simulink model "voter_logic_harness"  (Simulink 8.7)
settings: Solver=FixedStepDiscrete  StartTime=0  StopTime=1  FixedStep=1  RelTol=1e-3
undefined symbols (not defined in the file or in its folder): sigbuilder_block
libraries: sldvlib x10, simulink x6
settings Model: SldvGeneratedHarnessModel=TestUnitModel=voter_logic|
settings DataIOCC: SaveFormat=StructureWithTime
settings OptimizationCC: BlockReduction=off  ExpressionFolding=off
settings DebuggingCC: UnderspecifiedInitializationDetection=Simplified  MergeDetectMultiDrivingBlocksExec=error  InheritedTsInSrcMsg=none  AllowSymbolicDim=off
settings HardwareCC: ProdBitPerPointer=64  ProdLargestAtomicFloat=Float  ProdIntDivRoundTo=Zero  ProdEndianess=LittleEndian  ProdWordSize=64  ProdHWDeviceType=Intel->x86-64 (Windows64)
settings GRTTargetCC: GeneratePreprocessorConditionals=Use local settings
settings ConfigComp: CovModelRefEnable=off

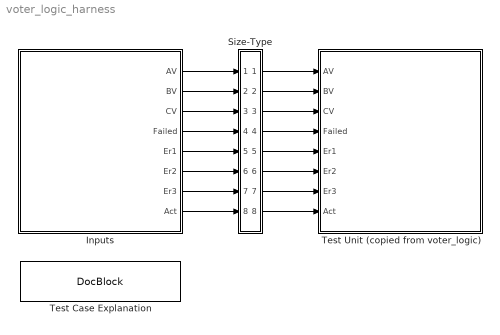
== system voter_logic_harness ==
  Inputs : Subsystem  Tag=STV Subsys  LoadFcn=sigbuilder_block('load',[459.75 78 519.75 399.75 ]);  StartFcn=sigbuilder_block('start');  StopFcn=sigbuilder_block('stop');  ClipboardFcn=sigbuilder_block('clipboard');  mask(Sigbuilder block){}
      mask init:
      | if ~strcmp(get_param(bdroot(gcb),'SimulationStatus'),'stopped'),tuvar = sigbuilder_block('maskInit'); end
      settings: CopyFcn=sigbuilder_block('copy');  DeleteFcn=sigbuilder_block('delete');  ModelCloseFcn=sigbuilder_block('modelClose');  PreSaveFcn=sigbuilder_block('preSave');  PauseFcn=sigbuilder_block('pause');  ContinueFcn=sigbuilder_block('continue');  NameChangeFcn=sigbuilder_block('namechange');  OpenFcn=sigbuilder_block('open');  CloseFcn=sigbuilder_block('close');
      mask Display: plot(0, 0, 100, 100,[2, 2, 32, 32, 2], [68, 8, 8, 68, 68],[32, 2], [38, 38], [32, 19, 2],[53, 60, 44], [32, 17, 17, 2],[16, 16, 31, 31]);txt = getActiveGroup(gcbh);text(2, 100, txt,'verticalAlignment', 'top');
  Size-Type : Subsystem
  Test Case Explanation : simulink/Model-Wide Utilities/DocBlock  DocumentType=Text
  Test Unit (copied from voter_logic) : Subsystem
  wires:
  Inputs/1(AV) -> Size-Type/1(In1)
  Size-Type/1(Out1) -> Test Unit (copied from voter_logic)/1(AV)
  Inputs/2(BV) -> Size-Type/2(In2)
  Size-Type/2(Out2) -> Test Unit (copied from voter_logic)/2(BV)
  Inputs/3(CV) -> Size-Type/3(In3)
  Size-Type/3(Out3) -> Test Unit (copied from voter_logic)/3(CV)
  Inputs/4(Failed) -> Size-Type/4(In4)
  Size-Type/4(Out4) -> Test Unit (copied from voter_logic)/4(Failed)
  Inputs/5(Er1) -> Size-Type/5(In5)
  Size-Type/5(Out5) -> Test Unit (copied from voter_logic)/5(Er1)
  Inputs/6(Er2) -> Size-Type/6(In6)
  Size-Type/6(Out6) -> Test Unit (copied from voter_logic)/6(Er2)
  Inputs/7(Er3) -> Size-Type/7(In7)
  Size-Type/7(Out7) -> Test Unit (copied from voter_logic)/7(Er3)
  Inputs/8(Act) -> Size-Type/8(In8)
  Size-Type/8(Out8) -> Test Unit (copied from voter_logic)/8(Act)

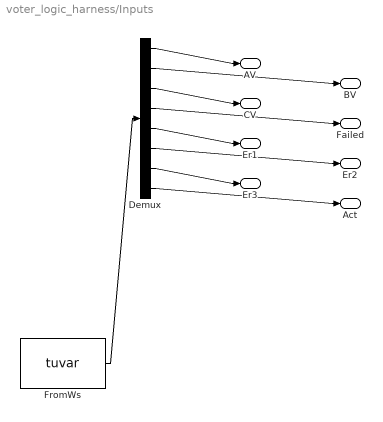
== system voter_logic_harness/Inputs ==
  Demux : Demux  Tag=STV Demux  Outputs=8
  FromWs : FromWorkspace  Tag=STV FromWs  VariableName=tuvar  SampleTime=0  SigBuilderData=DataTag0  VnvData=DataTag1
      SigBuilderData=|
      | dataSet.timeRange = [0 1]
      | dataSet.name = 'Counterexample 1'
      | sbobj.Name = 'Signal Builder'
      | sbobj.Groups.Name = 'Counterexample 1'
      | sbobj.Groups.Signals(1).Name = 'AV'
      | sbobj.Groups.Signals(1).XData = [0 1]
      | sbobj.Groups.Signals(1).YData = [1 1]
      | sbobj.Groups.Signals(2).Name = 'BV'
      | sbobj.Groups.Signals(2).XData = [0 1]
      | sbobj.Groups.Signals(2).YData = [0 0]
      | sbobj.Groups.Signals(3).Name = 'CV'
      | sbobj.Groups.Signals(3).XData = [0 1]
      | sbobj.Groups.Signals(3).YData = [1 1]
      | sbobj.Groups.Signals(4).Name = 'Failed'
      | sbobj.Groups.Signals(4).XData = [0 1]
      | sbobj.Groups.Signals(4).YData = [3 3]
      | sbobj.Groups.Signals(5).Name = 'Er1'
      | sbobj.Groups.Signals(5).XData = [0 1]
      | sbobj.Groups.Signals(5).YData = [-3 -3]
      | sbobj.Groups.Signals(6).Name = 'Er2'
      | sbobj.Groups.Signals(6).XData = [0 1]
      | sbobj.Groups.Signals(6).YData = [-3 -3]
      | sbobj.Groups.Signals(7).Name = 'Er3'
      | sbobj.Groups.Signals(7).XData = [0 1]
      | sbobj.Groups.Signals(7).YData = [-9 -9]
      | sbobj.Groups.Signals(8).Name = 'Act'
      | sbobj.Groups.Signals(8).XData = [0 1]
      | sbobj.Groups.Signals(8).YData = [60 60]
      | sbobj.Groups.TimeRange = [0 1]
  AV : Outport  Tag=STV Outport
  BV : Outport  Tag=STV Outport  Port=2
  CV : Outport  Tag=STV Outport  Port=3
  Failed : Outport  Tag=STV Outport  Port=4
  Er1 : Outport  Tag=STV Outport  Port=5
  Er2 : Outport  Tag=STV Outport  Port=6
  Er3 : Outport  Tag=STV Outport  Port=7
  Act : Outport  Tag=STV Outport  Port=8
  wires:
  FromWs/1 -> Demux/1
  Demux/1 -> AV/1
  Demux/2 -> BV/1
  Demux/3 -> CV/1
  Demux/4 -> Failed/1
  Demux/5 -> Er1/1
  Demux/6 -> Er2/1
  Demux/7 -> Er3/1
  Demux/8 -> Act/1

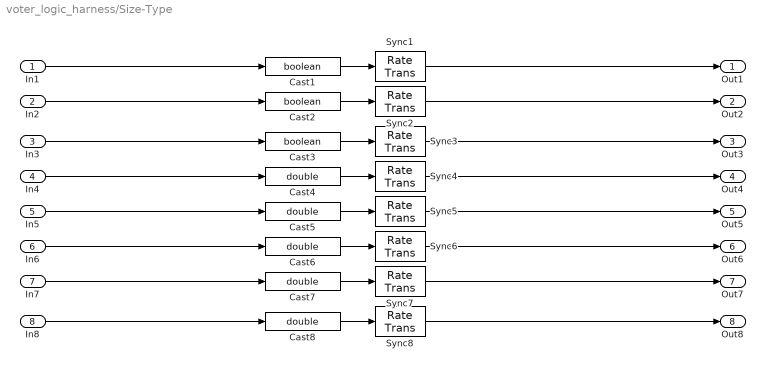
== system voter_logic_harness/Size-Type ==
  In1 : Inport
  In2 : Inport  Port=2
  In3 : Inport  Port=3
  In4 : Inport  Port=4
  In5 : Inport  Port=5
  In6 : Inport  Port=6
  In7 : Inport  Port=7
  In8 : Inport  Port=8
  Cast1 : DataTypeConversion  OutDataTypeStr=boolean  RndMeth=Nearest  SaturateOnIntegerOverflow=on
  Cast2 : DataTypeConversion  OutDataTypeStr=boolean  RndMeth=Nearest  SaturateOnIntegerOverflow=on
  Cast3 : DataTypeConversion  OutDataTypeStr=boolean  RndMeth=Nearest  SaturateOnIntegerOverflow=on
  Cast{4..8} (5 alike) : DataTypeConversion  OutDataTypeStr=double  RndMeth=Nearest  SaturateOnIntegerOverflow=on
  Sync{1..8} (8 alike) : RateTransition  OutPortSampleTime=[1,0]
  Out1 : Outport
  Out2 : Outport  Port=2
  Out3 : Outport  Port=3
  Out4 : Outport  Port=4
  Out5 : Outport  Port=5
  Out6 : Outport  Port=6
  Out7 : Outport  Port=7
  Out8 : Outport  Port=8
  wires:
  In1/1 -> Cast1/1
  Cast1/1 -> Sync1/1
  Sync1/1 -> Out1/1
  In2/1 -> Cast2/1
  Cast2/1 -> Sync2/1
  Sync2/1 -> Out2/1
  In3/1 -> Cast3/1
  Cast3/1 -> Sync3/1
  Sync3/1 -> Out3/1
  In4/1 -> Cast4/1
  Cast4/1 -> Sync4/1
  Sync4/1 -> Out4/1
  In5/1 -> Cast5/1
  Cast5/1 -> Sync5/1
  Sync5/1 -> Out5/1
  In6/1 -> Cast6/1
  Cast6/1 -> Sync6/1
  Sync6/1 -> Out6/1
  In7/1 -> Cast7/1
  Cast7/1 -> Sync7/1
  Sync7/1 -> Out7/1
  In8/1 -> Cast8/1
  Cast8/1 -> Sync8/1
  Sync8/1 -> Out8/1

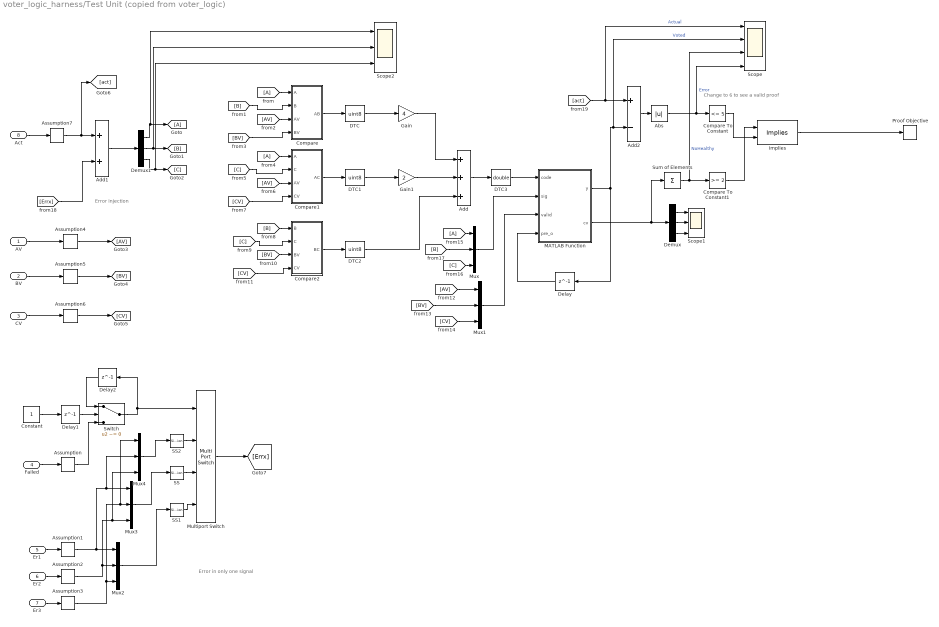
== system voter_logic_harness/Test Unit (copied from voter_logic) ==
  note: Change to 6 to see a valid proof
  note: Error in only one signal
  note: Error injection
  AV : Inport
  BV : Inport  Port=2
  CV : Inport  Port=3
  Failed : Inport  Port=4
  Er1 : Inport  Port=5
  Er2 : Inport  Port=6
  Er3 : Inport  Port=7
  Act : Inport  Port=8
  Abs : Abs
  Add : Sum  Inputs=+++
  Add1 : Sum
  Add2 : Sum  Inputs=+-
  Assumption : sldvlib/Objectives and Constraints/Assumption  enabled=on  customAVTBlockType=Assumption  intervals={1,2,3}  initial=off  dispValues=on  outEnabled=on
      settings: AttributesFormatString=%<intervals>
  Assumption1 : sldvlib/Objectives and Constraints/Assumption  enabled=on  customAVTBlockType=Assumption  intervals={[-3 3]}  initial=off  dispValues=on  outEnabled=on
      settings: AttributesFormatString=%<intervals>
  Assumption2 : sldvlib/Objectives and Constraints/Assumption  enabled=on  customAVTBlockType=Assumption  intervals={[-3 3]}  initial=off  dispValues=on  outEnabled=on
      settings: AttributesFormatString=%<intervals>
  Assumption3 : sldvlib/Objectives and Constraints/Assumption  enabled=on  customAVTBlockType=Assumption  intervals="{[-40  40]}"  initial=off  dispValues=on  outEnabled=on
      settings: AttributesFormatString=%<intervals>
  Assumption4 : sldvlib/Objectives and Constraints/Assumption  enabled=on  customAVTBlockType=Assumption  intervals={0,1}  initial=off  dispValues=on  outEnabled=on
      settings: AttributesFormatString=%<intervals>
  Assumption5 : sldvlib/Objectives and Constraints/Assumption  enabled=on  customAVTBlockType=Assumption  intervals={0,1}  initial=off  dispValues=on  outEnabled=on
      settings: AttributesFormatString=%<intervals>
  Assumption6 : sldvlib/Objectives and Constraints/Assumption  enabled=on  customAVTBlockType=Assumption  intervals={0,1}  initial=off  dispValues=on  outEnabled=on
      settings: AttributesFormatString=%<intervals>
  Assumption7 : sldvlib/Objectives and Constraints/Assumption  enabled=on  customAVTBlockType=Assumption  intervals={[60 300]}  initial=off  dispValues=on  outEnabled=on
      settings: AttributesFormatString=%<intervals>
  Compare : Subsystem
  Compare To Constant : simulink/Logic and Bit Operations/Compare To Constant  relop=<=  const=5  OutDataTypeStr=boolean
  Compare To Constant1 : simulink/Logic and Bit Operations/Compare To Constant  relop=>=  const=2  OutDataTypeStr=boolean
  Compare1 : Subsystem
  Compare2 : Subsystem
  Constant : Constant
  DTC : DataTypeConversion  OutDataTypeStr=uint8
  DTC1 : DataTypeConversion  OutDataTypeStr=uint8
  DTC2 : DataTypeConversion  OutDataTypeStr=uint8
  DTC3 : DataTypeConversion  OutDataTypeStr=double
  Delay : Delay  DelayLength=1  InitialCondition=0
  Delay1 : Delay  DelayLength=1  InitialCondition=0
  Delay2 : Delay  DelayLength=1  InitialCondition=0
  Demux : Demux  Outputs=3
  Demux1 : Demux  Outputs=3
  Gain : Gain  Gain=4
  Gain1 : Gain  Gain=2
  Implies : sldvlib/Verification Utilities/Implies
  MATLAB Function : MATLAB Function  TreatAsAtomicUnit=on
  Multiport Switch : MultiPortSwitch
  Mux{,1..4} (5 alike) : Mux  Inputs=3
  Proof Objective : sldvlib/Objectives and Constraints/Proof Objective  enabled=on  customAVTBlockType=Proof Objective  intervals=true  dispValues=on  outEnabled=off  enableStopSim=off
      settings: AttributesFormatString=%<intervals>
  SS : SignalSpecification  Dimensions=3
  SS1 : SignalSpecification  Dimensions=3
  SS2 : SignalSpecification  Dimensions=3
  Scope : Scope  NumInputPorts=4
  Scope1 : Scope  NumInputPorts=3
  Scope2 : Scope  NumInputPorts=3
  Sum of Elements : Sum  Inputs=+
  Switch : Switch  Criteria=u2 ~= 0
  wires:
  Compare/1(AB) -> DTC/1
  Compare1/1(AC) -> DTC1/1
  Compare2/1(BC) -> DTC2/1
  DTC/1 -> Gain/1
  DTC1/1 -> Gain1/1
  Gain/1 -> Add/1
  Gain1/1 -> Add/2
  DTC2/1 -> Add/3
  AV/1 -> Assumption4/1
  BV/1 -> Assumption5/1
  CV/1 -> Assumption6/1
  [A] -> Compare/1(A)
  [B] -> Compare/2(B)
  [AV] -> Compare/3(AV)
  [BV] -> Compare/4(BV)
  [A] -> Compare1/1(A)
  [C] -> Compare1/2(C)
  [AV] -> Compare1/3(AV)
  [CV] -> Compare1/4(CV)
  [B] -> Compare2/1(B)
  [C] -> Compare2/2(C)
  [BV] -> Compare2/3(BV)
  [CV] -> Compare2/4(CV)
  Add/1 -> DTC3/1
  Delay/1 -> MATLAB Function/4(pre_o)
  MATLAB Function/1(y) -> Delay/1, Add2/2, Scope/2  "Voted"
  Mux/1 -> MATLAB Function/2(sig)
  Mux1/1 -> MATLAB Function/3(valid)
  [AV] -> Mux1/1
  [BV] -> Mux1/2
  [CV] -> Mux1/3
  [A] -> Mux/1
  [B] -> Mux/2
  [C] -> Mux/3
  MATLAB Function/2(cv) -> Demux/1, Sum of Elements/1
  Demux1/2 -> Scope2/2, [B]
  Demux1/1 -> Scope2/1, [A]
  Demux1/3 -> Scope2/3, [C]
  Add1/1 -> Demux1/1
  [Errx] -> Add1/2
  Delay1/1 -> Switch/2
  Constant/1 -> Delay1/1
  Switch/1 -> Multiport Switch/1, Delay2/1
  Failed/1 -> Assumption/1
  Assumption/1 -> Switch/3
  Er1/1 -> Assumption1/1
  Er2/1 -> Assumption2/1
  Er3/1 -> Assumption3/1
  Multiport Switch/1 -> [Errx]
  Delay2/1 -> Switch/1
  Assumption4/1 -> [AV]
  Assumption5/1 -> [BV]
  Assumption6/1 -> [CV]
  Act/1 -> Assumption7/1
  Assumption7/1 -> Add1/1, [act]
  [act] -> Add2/1, Scope/1  "Actual"
  Add2/1 -> Abs/1
  Abs/1 -> Compare To Constant/1, Scope/4  "Error"
  SS/1 -> Multiport Switch/3
  SS1/1 -> Multiport Switch/4
  SS2/1 -> Multiport Switch/2
  DTC3/1 -> MATLAB Function/1(code)
  Sum of Elements/1 -> Scope/3, Compare To Constant1/1  "NoHealthy"
  Compare To Constant1/1 -> Implies/1
  Compare To Constant/1 -> Implies/2
  Implies/1 -> Proof Objective/1
  Assumption1/1 -> Mux2/1, Mux3/1, Mux4/2
  Assumption2/1 -> Mux2/2, Mux3/3, Mux4/3
  Assumption3/1 -> Mux2/3, Mux3/2, Mux4/1
  Mux2/1 -> SS1/1
  Mux3/1 -> SS/1
  Mux4/1 -> SS2/1
  Demux/1 -> Scope1/1
  Demux/2 -> Scope1/2
  Demux/3 -> Scope1/3

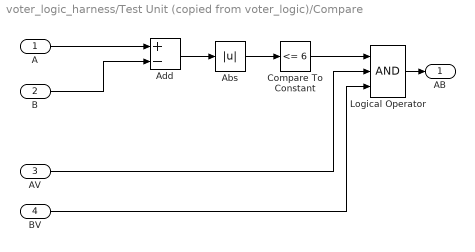
== system voter_logic_harness/Test Unit (copied from voter_logic)/Compare ==
  A : Inport
  B : Inport  Port=2
  AV : Inport  Port=3
  BV : Inport  Port=4
  Abs : Abs
  Add : Sum  Inputs=+-
  Compare To Constant : simulink/Logic and Bit Operations/Compare To Constant  relop=<=  const=6  OutDataTypeStr=boolean
  Logical Operator : Logic  Inputs=3  AllPortsSameDT=off  OutDataTypeStr=boolean
  AB : Outport
  wires:
  Logical Operator/1 -> AB/1
  Add/1 -> Abs/1
  BV/1 -> Logical Operator/3
  A/1 -> Add/1
  AV/1 -> Logical Operator/2
  B/1 -> Add/2
  Abs/1 -> Compare To Constant/1
  Compare To Constant/1 -> Logical Operator/1

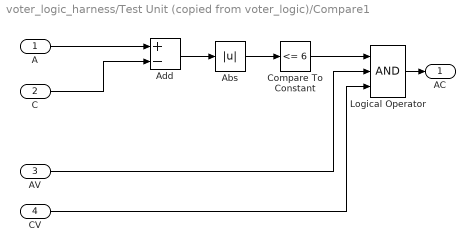
== system voter_logic_harness/Test Unit (copied from voter_logic)/Compare1 ==
  A : Inport
  C : Inport  Port=2
  AV : Inport  Port=3
  CV : Inport  Port=4
  Abs : Abs
  Add : Sum  Inputs=+-
  Compare To Constant : simulink/Logic and Bit Operations/Compare To Constant  relop=<=  const=6  OutDataTypeStr=boolean
  Logical Operator : Logic  Inputs=3  AllPortsSameDT=off  OutDataTypeStr=boolean
  AC : Outport
  wires:
  Compare To Constant/1 -> Logical Operator/1
  Abs/1 -> Compare To Constant/1
  C/1 -> Add/2
  AV/1 -> Logical Operator/2
  A/1 -> Add/1
  CV/1 -> Logical Operator/3
  Add/1 -> Abs/1
  Logical Operator/1 -> AC/1

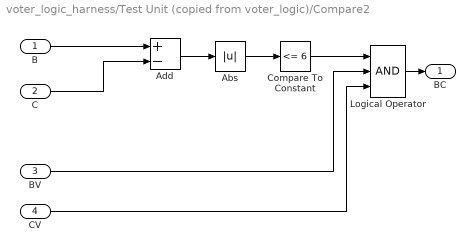
== system voter_logic_harness/Test Unit (copied from voter_logic)/Compare2 ==
  B : Inport
  C : Inport  Port=2
  BV : Inport  Port=3
  CV : Inport  Port=4
  Abs : Abs
  Add : Sum  Inputs=+-
  Compare To Constant : simulink/Logic and Bit Operations/Compare To Constant  relop=<=  const=6  OutDataTypeStr=boolean
  Logical Operator : Logic  Inputs=3  AllPortsSameDT=off  OutDataTypeStr=boolean
  BC : Outport
  wires:
  Logical Operator/1 -> BC/1
  Add/1 -> Abs/1
  CV/1 -> Logical Operator/3
  B/1 -> Add/1
  BV/1 -> Logical Operator/2
  C/1 -> Add/2
  Abs/1 -> Compare To Constant/1
  Compare To Constant/1 -> Logical Operator/1

== matlab function Test Unit (copied from voter_logic)/MATLAB Function ==
  data: code input double; y output double; sig input double; valid input double; pre_o input double; cv output double
function [y, cv] = fcn(code,sig,valid,pre_o)
%#codegen
% AB   AC   BC  
%  0    0    0      (0) All fail
%  0    0    1      (1) A fail
%  0    1    0      (2) B fail
%  0    1    1      (3) C valid
%  1    0    0      (4) C fail
%  1    0    1      (5) B valid
%  1    1    0      (6) A valid
%  1    1    1      (7) All valid

cv = zeros(3,1);
y=0;
if code == 0
    y = pre_o;
    cv = [0;0;0];    % all fail hold prev value
elseif code == 1
    y = (sig(2)+sig(3))/2;
    cv = [0;1;1];     % A fail use average of B C
elseif code == 2
    y = (sig(1)+sig(3))/2;
    cv = [1;0;1];  % B fail use average A C
elseif code == 3
    y = sig(3);
    cv = [valid(1);valid(2);1]; % C valid
elseif code == 4
    y = (sig(1)+sig(2))/2;
    cv = [1;1;0];  % C fail use average A B
elseif code == 5
    y = sig(2);
    cv = [valid(1);1;valid(3)]; % B valid
elseif code == 6
    y = sig(1);
    cv = [1;valid(2);valid(3)]; % A valid
elseif code == 7
    y = (sig(1)+sig(2)+sig(3))/3;
    cv = [1;1;1]; % All valid
end
